simulink model "H4Q_FPGA"  (Simulink 8.1)
settings: Solver=ode3  SolverMode=SingleTasking  StartTime=0.0  StopTime=0.9  FixedStep=Ts  RelTol=1e-3
PostLoadFcn:
  | Init_Params;
InitFcn:
  | Init_Params;
values from neighbouring files (symbols this model uses):
  L = .1    (= 0.1)    [Init_Params.m]
  R = .28    (= 0.28)    [Init_Params.m]
  Tpas = Ts    (= 2.5e-05)    [Init_Params.m]
libraries: powerlib x10, rteventslib x1
settings Model: Creator=LiberT  LastModifiedBy=Francis
settings DebuggingCC: MultiTaskDSMMsg=warning  MultiTaskCondExecSysMsg=none  FcnCallInpInsideContextMsg=EnableAllAsWarning  UnconnectedInputMsg=none  UnconnectedOutputMsg=none  UnconnectedLineMsg=none  StrictBusMsg=None
settings RTWCC: IncludeERTFirstTime=on

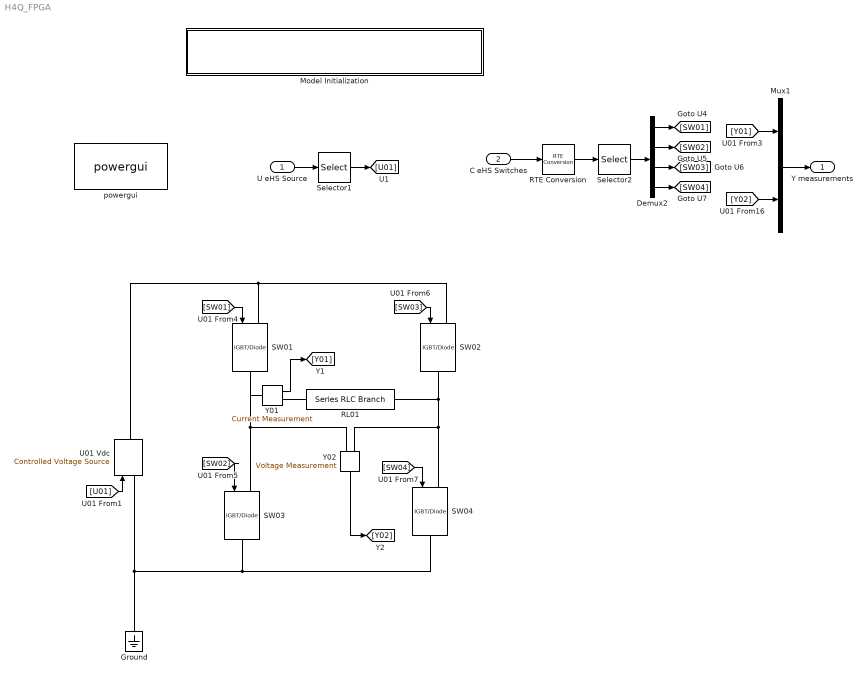
== system H4Q_FPGA ==
  U eHS Source : Inport
  C eHS Switches : Inport  Port=2
  Demux2 : Demux
  Ground : powerlib/Elements/Ground  LConnTagsString=a
  Model Initialization : Subsystem  mask(Model Functions){InitFcnX=Init_Params;, prel=off, posl=on, inif=on, strf=off}
      mask prompts: InitFcnX "Initialisation"; prel "Preload Function"; posl "PostLoad Function"; inif "InitFcn"; strf "StartFcn"
      mask init:
      | currentBlock = gcb;
      | root = bdroot(currentBlock);
      | 
      | if ~strcmp(get_param(root,'BlockDiagramType'),'library')
      |     if prel==1
      |         set_param(root, 'PreLoadFcn', InitFcnX);
      |     else
      |         set_param(root, 'PreLoadFcn', '');
      |     end
      |     if inif==1
      |         set_param(root, 'InitFcn', InitFcnX);
      |     else
      |         set_param(root, 'InitFcn', '');
      |     end
      |     if strf==1
      |         set_param(root, 'StartFcn', InitFcnX);
      |     else
      |         set_param(root, 'StartFcn', '');
      |     end
      |     if posl==1
      |         set_param(root, 'PostLoadFcn', InitFcnX);
      |     else
      |         set_param(root, 'PostLoadFcn', '');
      |     end
      | end
      | 
      | pos = get_param(currentBlock, 'Position');
      | width = pos(3) - pos(1); height = pos(4) - pos(2);
      | txt = [ upper(root) '\n' '- InitFcn. . . . . '  get_param(root, 'InitFcn') ];
      settings: CopyFcn=set_param(gcb,'LinkStatus','none')
      mask Display: text(5, height*0.5, txt, 'horizontalAlignment', 'left', 'verticalAlignment', 'middle') ;
  Mux1 : Mux  Inputs=2
  RL01 : powerlib/Elements/Series RLC Branch  LConnTagsString=__new0  RConnTagsString=__new0  BranchType=RL  Resistance=R  Inductance=L  SetiL0=off  InitialCurrent=0  Capacitance=2000e-6  Setx0=off  InitialVoltage=0  Measurements=None
  RTE Conversion : rteventslib/Signal Attributes/RTE Conversion  inputdatatype=RTE Boolean  outputdatatype=Double  compensation=Enabled  nbMaxEvents=2  sampleTime=Ts
  SW01 : powerlib/Power Electronics/IGBT//Diode  Ron=GsR  Rs=1e5  Cs=inf  Measurements=off
  SW02 : powerlib/Power Electronics/IGBT//Diode  Ron=GsR  Rs=1e5  Cs=inf  Measurements=off
  SW03 : powerlib/Power Electronics/IGBT//Diode  Ron=GsR  Rs=1e5  Cs=inf  Measurements=off
  SW04 : powerlib/Power Electronics/IGBT//Diode  Ron=GsR  Rs=1e5  Cs=inf  Measurements=off
  Selector1 : Selector  IndexOptions=Index vector (dialog)  Indices=[1]  OutputSizes=1
  Selector2 : Selector  IndexOptions=Index vector (dialog)  Indices=[1:4]  OutputSizes=1
  U01 Vdc : powerlib/Electrical Sources/Controlled Voltage Source  Initialize=off  Source_Type=AC  Amplitude=0  Phase=0  Frequency=0  Measurements=None
  Y01 : powerlib/Measurements/Current Measurement  PhasorSimulation=off  OutputType=Complex  PSBequivalent=0
  Y02 : powerlib/Measurements/Voltage Measurement  PhasorSimulation=off  OutputType=Complex  PSBequivalent=0
  powergui : powerlib/powergui  Priority=1  SimulationMode=Continuous  SolverType=Tustin  SampleTime=Tpas  frequency=60  SPID=off  DisableSnubberDevices=off  DisableRonSwitches=off  DisableVfSwitches=off  SwTol=0  Interpol=off  DisplayEquations=off  frequencyindice=0  Pbase=100e6  ErrMax=1e-4  Iterations=50  UnitsV=kV  UnitsW=MW  FunctionMessages=off  echomessages=off  HookPort=off  EnableUseOfTLC=off  x0status=blocks  RestoreLinks=warning  ResistiveCurrentMeasurement=off  Frange=[0:2:500]  Ylog=off  Xlog=on  ShowGrid=off  save=off  variable=ZData  structure=ScopeData  ZoomFFT=off  StartTime=7.29  cycles=3  DisplayStyle=1  fundamental=50  FreqAxis=off  MaxFrequency=1000  frequencyindicesteady=1  RmsSteady=1  display=off  Ts=0  methode=off
  Y measurements : Outport
  wires:
  [SW01] -> SW01/1
  [U01] -> U01 Vdc/1
  [SW02] -> SW03/1
  [SW03] -> SW02/1
  [SW04] -> SW04/1
  Demux2/4 -> [SW04]
  Demux2/3 -> [SW03]
  Demux2/2 -> [SW02]
  Demux2/1 -> [SW01]
  C eHS Switches/1 -> RTE Conversion/1
  Mux1/1 -> Y measurements/1
  U eHS Source/1 -> Selector1/1
  [Y01] -> Mux1/1
  [Y02] -> Mux1/2
  Selector1/1 -> [U01]
  Selector2/1 -> Demux2/1
  RTE Conversion/1 -> Selector2/1
  Y01/1 -> [Y01]
  Y02/1 -> [Y02]
  connections:
  SW01/RConn1 -- Y01/LConn1 -- SW03/LConn1 -- Y02/LConn1
  SW02/RConn1 -- SW04/LConn1 -- Y02/LConn2 -- RL01/LConn1
  SW03/RConn1 -- SW04/RConn1 -- Ground/LConn1 -- U01 Vdc/LConn1
  SW02/LConn1 -- SW01/LConn1 -- U01 Vdc/RConn1
  Y01/RConn1 -- RL01/RConn1

== system H4Q_FPGA/Model Initialization ==
